simulink model "lab_11"  (R2020b)
settings: Solver=VariableStepAuto  StartTime=0.0  StopTime=100  RelTol=1e-3
libraries: simulink x1, simulink_extras x1
settings Model: Creator=pawel  LastModifiedBy=pawel

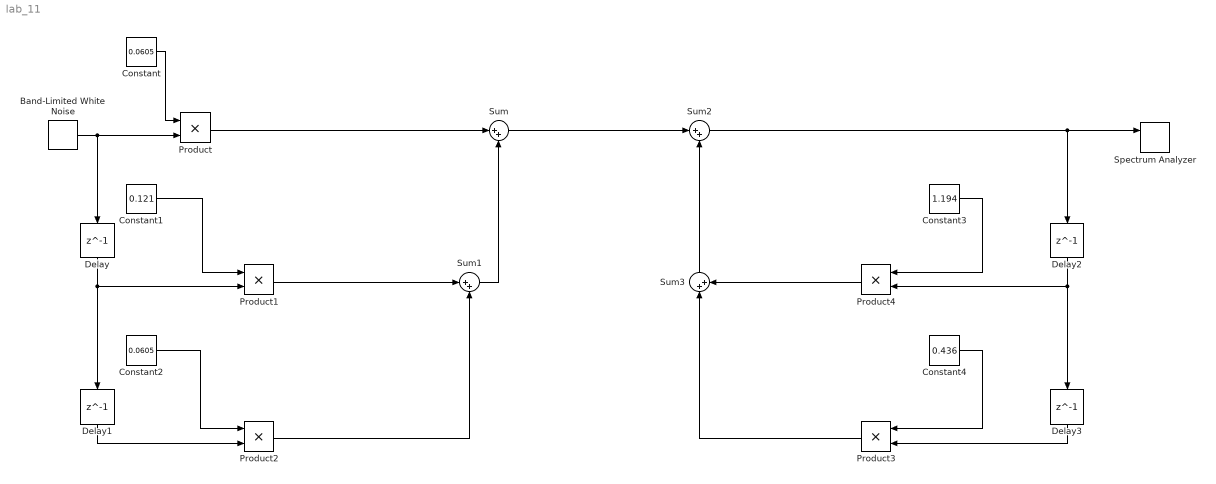
== system lab_11 ==
  Band-Limited White Noise : simulink/Sources/Band-Limited White Noise  Cov=[0.1]  Ts=1/10000  seed=[23341]
  Constant : Constant  Value=0.0605
  Constant1 : Constant  Value=0.121
  Constant2 : Constant  Value=0.0605
  Constant3 : Constant  Value=1.194
  Constant4 : Constant  Value=0.436
  Delay{,1..3} (4 alike) : Delay  DelayLength=1  InitialCondition=0
  Product{,1..4} (5 alike) : Product
  Spectrum Analyzer : simulink_extras/Additional Sinks/Spectrum Analyzer  npts=256  fftpts=256  HowOften=64  sampleT=0.1
      settings: SourceProductBaseCode=SL
  Sum{,1..3} (4 alike) : Sum  Inputs=|++
  wires:
  Constant/1 -> Product/1
  Band-Limited White Noise/1 -> Product/2, Delay/1
  Product/1 -> Sum/1
  Constant1/1 -> Product1/1
  Product1/1 -> Sum1/1
  Product2/1 -> Sum1/2
  Sum1/1 -> Sum/2
  Sum/1 -> Sum2/1
  Sum3/1 -> Sum2/2
  Delay/1 -> Delay1/1, Product1/2
  Delay1/1 -> Product2/2
  Constant2/1 -> Product2/1
  Sum2/1 -> Spectrum Analyzer/1, Delay2/1
  Delay2/1 -> Product4/2, Delay3/1
  Delay3/1 -> Product3/2
  Product4/1 -> Sum3/2
  Product3/1 -> Sum3/1
  Constant4/1 -> Product3/1
  Constant3/1 -> Product4/1
